simulink model "gcfc"  (R2021a)
settings: Solver=VariableStepAuto  StartTime=0.0  StopTime=15000  RelTol=1e-3
values from neighbouring files (symbols this model uses):
  Ts = 0.5    [Distillation_Column_model_identification.m]    (also in Distillation_Column_model_variance.m; fourvary.m = 8)
libraries: dspsrcs4 x1
settings Model: Creator=dell  LastModifiedBy=dell

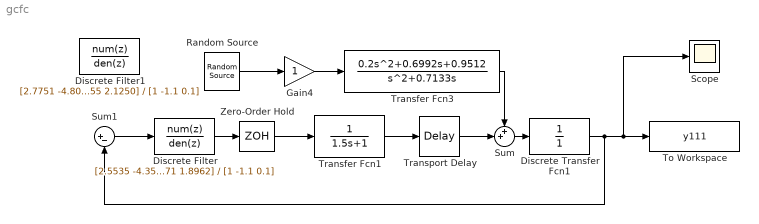
== system gcfc ==
  Discrete Transfer Fcn1 : DiscreteTransferFcn  Denominator=[1]  SampleTime=Ts
      mask Display: disp('sampler')
  Discrete Filter : DiscreteFilter  Numerator=[2.5535 -4.3571 1.8962]  Denominator=[1 -1.1 0.1]  SampleTime=Ts
  Discrete Filter1 : DiscreteFilter  Numerator=[2.7751 -4.8055 2.1250]  Denominator=[1 -1.1 0.1]  SampleTime=Ts
  Gain4 : Gain
  Random Source : dspsrcs4/Random Source  SrcType=Gaussian  NormMethod=Ziggurat  CltLength=12  MinVal=-1  MaxVal=1  MeanVal=0  VarVal=1  RepMode=Specify seed  rawSeed=1  IsInherit=off  SampMode=Continuous  SampTime=1  SampFrame=1  DataType=Double  OutComplex=Real  OutputFrames=off
  Scope : Scope
  Sum : Sum  Inputs=++|
  Sum1 : Sum  Inputs=|+-
  To Workspace : ToWorkspace  VariableName=y111  SampleTime=Ts
  Transfer Fcn1 : TransferFcn  Denominator=[1.5 1]
  Transfer Fcn3 : TransferFcn  Numerator=[0.2 0.6992 0.9512]  Denominator=[1 0.7133 0]
  Transport Delay : TransportDelay  DelayTime=5
  Zero-Order Hold : ZeroOrderHold  SampleTime=Ts
  wires:
  Sum/1 -> Discrete Transfer Fcn1/1
  Zero-Order Hold/1 -> Transfer Fcn1/1
  Gain4/1 -> Transfer Fcn3/1
  Random Source/1 -> Gain4/1
  Transport Delay/1 -> Sum/2
  Transfer Fcn1/1 -> Transport Delay/1
  Sum1/1 -> Discrete Filter/1
  Transfer Fcn3/1 -> Sum/1
  Discrete Transfer Fcn1/1 -> Sum1/2, Scope/1, To Workspace/1
  Discrete Filter/1 -> Zero-Order Hold/1
